simulink model "ii_270degree"  (R2023a)
settings: Solver=FixedStepDiscrete  StartTime=0.0  StopTime=30  FixedStep=0.01  RelTol=1e-3
values from neighbouring files (symbols this model uses):
  axleLength = 0.136    [robotParameters.m]
  ticksPerRot = 10    [robotParameters.m]
  wheelR = 0.034    [robotParameters.m]
undefined symbols (not defined in the file or in its folder): InputPWM, WheelSpeed
libraries: mobileRoboticsTrainingLib x5, simulink x1
settings Model: Creator=Boitumelo  LastModifiedBy=cameronclark
settings DebuggingCC: UnconnectedInputMsg=warning  UnconnectedOutputMsg=warning  UnconnectedLineMsg=warning
settings ModelReferenceCC: EnableRefExpFcnMdlSchedulingChecks=on
settings RTWCC: DLArmComputeVersion=19.05

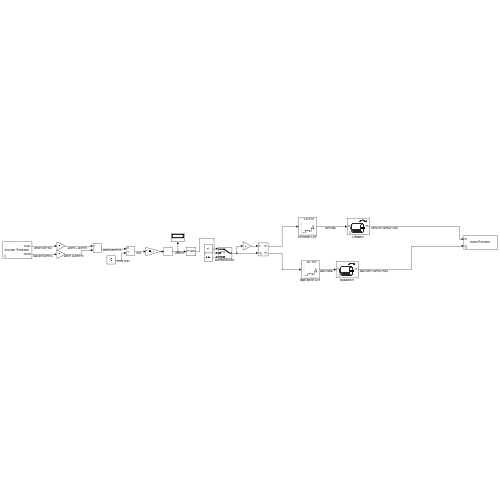
[thumbnail: Simulink's stored preview of the top-level diagram]
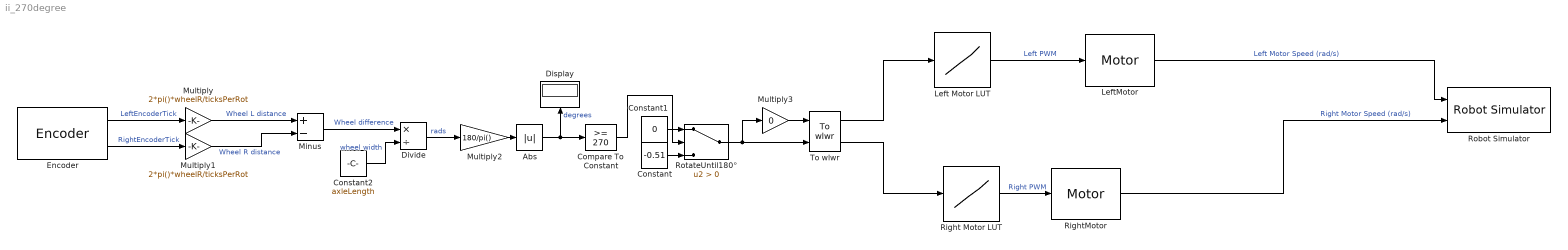
== system ii_270degree ==
  Abs : Abs  SaturateOnIntegerOverflow=off
  Compare To Constant : simulink/Logic and Bit Operations/Compare To Constant  relop=>=  const=270  OutDataTypeStr=boolean
  Constant : Constant  Value=-0.51
  Constant1 : Constant  Value=0
  Constant2 : Constant  Value=axleLength
  Display : Display
  Divide : Product  Inputs=*/
  Encoder : mobileRoboticsTrainingLib/Encoder  axleLength=axleLength  wheelR=wheelR  ticksPerRot=ticksPerRot
      settings: SourceProductName=Mobile Robotics Training Library
  Left Motor LUT : Lookup_n-D  NumberOfTableDimensions=1  BreakpointsForDimension1=WheelSpeed  Table=InputPWM  InterpMethod=Nearest  ExtrapMethod=Clip  InternalRulePriority=Speed  RndMeth=Simplest
  LeftMotor : mobileRoboticsTrainingLib/Motor  motorPlant=wheelMotorModel  sensorType=Speed
      settings: SourceProductName=Mobile Robotics Training Library
  Minus : Sum  Inputs=+-
  Multiply : Gain  Gain=2*pi()*wheelR/ticksPerRot
  Multiply1 : Gain  Gain=2*pi()*wheelR/ticksPerRot
  Multiply2 : Gain  Gain=180/pi()
  Multiply3 : Gain  Gain=0
  Right Motor LUT : Lookup_n-D  NumberOfTableDimensions=1  BreakpointsForDimension1=WheelSpeed  Table=InputPWM  InterpMethod=Nearest  ExtrapMethod=Clip  InternalRulePriority=Speed  RndMeth=Simplest
  RightMotor : mobileRoboticsTrainingLib/Motor  motorPlant=wheelMotorModel  sensorType=Speed
      settings: SourceProductName=Mobile Robotics Training Library
  Robot Simulator : mobileRoboticsTrainingLib/Robot Simulator  Priority=99  mapVar=mapForSim  startX=0.2  startY=0.2  startTheta=90  axleLength=axleLength  wheelR=wheelR
  RotateUntil180° : Switch  Criteria=u2 > Threshold  SaturateOnIntegerOverflow=off  InputSameDT=off
  To wlwr : mobileRoboticsTrainingLib/To wlwr  axleLength=0.1  wheelR=0.05
  wires:
  Right Motor LUT/1 -> RightMotor/1  "Right PWM"
  Left Motor LUT/1 -> LeftMotor/1  "Left PWM"
  To wlwr/1 -> Left Motor LUT/1
  To wlwr/2 -> Right Motor LUT/1
  RightMotor/1 -> Robot Simulator/2  "Right Motor Speed (rad/s)"
  LeftMotor/1 -> Robot Simulator/1  "Left Motor Speed (rad/s)"
  Multiply3/1 -> To wlwr/1
  Constant/1 -> RotateUntil180°/3
  Divide/1 -> Multiply2/1  "rads"
  Encoder/1 -> Multiply/1  "LeftEncoderTick"
  RotateUntil180°/1 -> To wlwr/2, Multiply3/1
  Constant2/1 -> Divide/2  "wheel width"
  Compare To Constant/1 -> RotateUntil180°/2
  Multiply/1 -> Minus/1  "Wheel L distance"
  Multiply2/1 -> Abs/1
  Minus/1 -> Divide/1  "Wheel difference"
  Constant1/1 -> RotateUntil180°/1
  Multiply1/1 -> Minus/2  "Wheel R distance"
  Encoder/2 -> Multiply1/1  "RightEncoderTick"
  Abs/1 -> Compare To Constant/1, Display/1  "degrees"
